simulink model "control_system"  (R2020a)
settings: Solver=VariableStepAuto  StartTime=0.0  StopTime=1000  RelTol=1e-3
InitFcn:
  | LAB2
values from neighbouring files (symbols this model uses):
  A = [-0.342 0 0.0318; 0 -0.0716 0.0318; 0.0204 0.0204 -0.0423]    [LAB2.m]
  B = [0.159 0; 0 0.159; 0 0]    [LAB2.m]
  K = K_(:,1:3)    [LAB2.m]
  N = K_(:,4:end)    [LAB2.m]
settings Model: Creator=paulogil  LastModifiedBy=joaom
settings OptimizationCC: LifeSpan=inf
settings DebuggingCC: SFExecutionAtInitializationDiag=none  ArithmeticOperatorsInVariantConditions=warning
settings SFSimCC: CustomCodeUndefinedFunction=UseInterfaceOnly
settings CodeAppCC: StateflowObjectComments=on

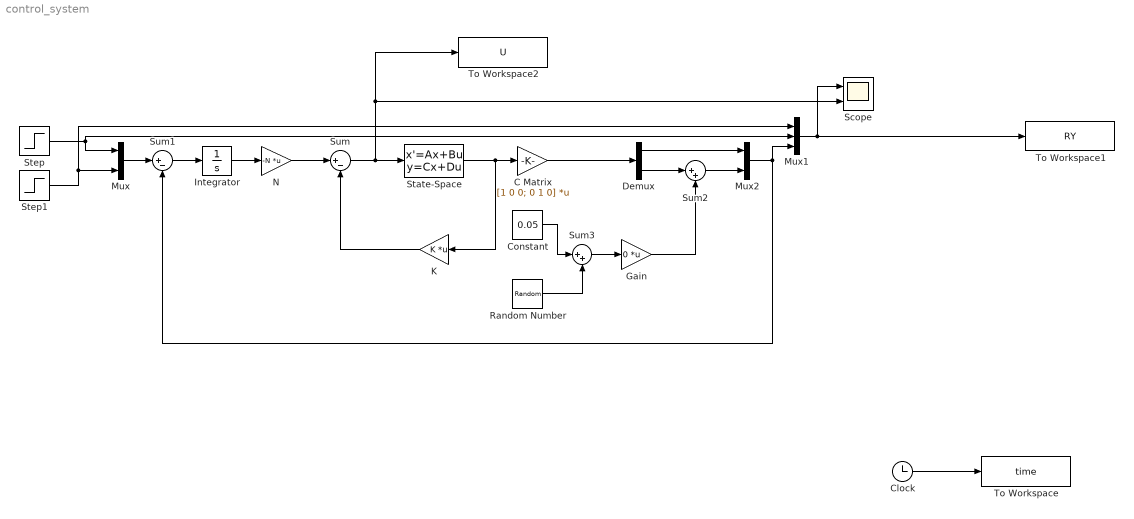
== system control_system ==
  C Matrix : Gain  Gain=[1 0 0; 0 1 0]  Multiplication=Matrix(K*u)
  Clock : Clock
  Constant : Constant  Value=0.05
  Demux : Demux  Outputs=2
  Gain : Gain  Gain=0  Multiplication=Matrix(K*u)
  Integrator : Integrator
  K : Gain  Gain=K  Multiplication=Matrix(K*u)
  Mux : Mux  Inputs=2
  Mux1 : Mux  Inputs=3
  Mux2 : Mux  Inputs=2
  N : Gain  Gain=-N  Multiplication=Matrix(K*u)
  Random Number : RandomNumber  Variance=0.001  SampleTime=0.1
  Scope : Scope  NumInputPorts=2
  State-Space : StateSpace  A=A  B=B  C=eye(3)  D=zeros(3,2)  InitialCondition=0
  Step : Step  Time=0  After=0.5  SampleTime=0
  Step1 : Step  After=0.7  SampleTime=0
  Sum : Sum  Inputs=|+-
  Sum1 : Sum  Inputs=|+-
  Sum2 : Sum  Inputs=|++
  Sum3 : Sum  Inputs=|++
  To Workspace : ToWorkspace  VariableName=time  SaveFormat=Timeseries  SampleTime=-1
  To Workspace1 : ToWorkspace  VariableName=RY  SaveFormat=Timeseries  SampleTime=-1
  To Workspace2 : ToWorkspace  VariableName=U  SaveFormat=Timeseries  SampleTime=-1
  wires:
  State-Space/1 -> K/1, C Matrix/1
  K/1 -> Sum/2
  N/1 -> Sum/1
  Mux1/1 -> To Workspace1/1, Scope/1
  Clock/1 -> To Workspace/1
  Integrator/1 -> N/1
  Sum1/1 -> Integrator/1
  Step/1 -> Mux1/2, Mux/1
  Step1/1 -> Mux1/1, Mux/2
  Mux/1 -> Sum1/1
  Constant/1 -> Sum3/1
  Sum3/1 -> Gain/1
  Random Number/1 -> Sum3/2
  Gain/1 -> Sum2/2
  C Matrix/1 -> Demux/1
  Demux/2 -> Sum2/1
  Sum2/1 -> Mux2/2
  Demux/1 -> Mux2/1
  Mux2/1 -> Sum1/2, Mux1/3
  Sum/1 -> To Workspace2/1, Scope/2, State-Space/1
